simulink model "reguladores"  (R2019a)
settings: Solver=VariableStepAuto  StartTime=0.0  StopTime=10.0  RelTol=1e-3
undefined symbols (not defined in the file): Kregulador
settings Model: Creator=julia  LastModifiedBy=julia

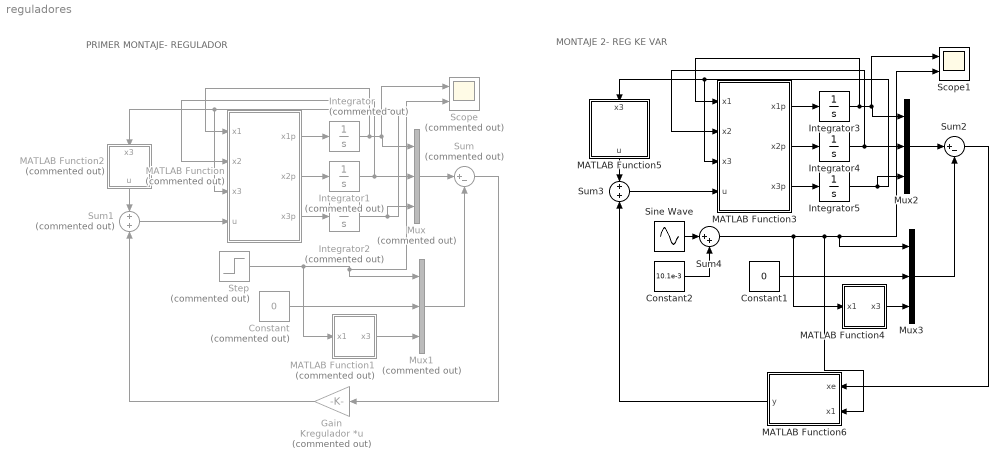
== system reguladores ==
  note: MONTAJE 2- REG KE VAR
  note: PRIMER MONTAJE- REGULADOR
  Constant : Constant  Commented=on  Value=0
  Constant1 : Constant  Value=0
  Constant2 : Constant  Value=10.1e-3
  Gain : Gain  Commented=on  Gain=Kregulador  Multiplication=Matrix(K*u)
  Integrator : Integrator  Commented=on  InitialCondition=5e-3
  Integrator1 : Integrator  Commented=on
  Integrator2 : Integrator  Commented=on
  Integrator3 : Integrator  InitialCondition=5e-3
  Integrator4 : Integrator
  Integrator5 : Integrator
  MATLAB Function : MATLAB Function  Commented=on  TreatAsAtomicUnit=on
  MATLAB Function1 : MATLAB Function  Commented=on  TreatAsAtomicUnit=on
  MATLAB Function2 : MATLAB Function  Commented=on  TreatAsAtomicUnit=on
  MATLAB Function3 : MATLAB Function  TreatAsAtomicUnit=on
  MATLAB Function4 : MATLAB Function  TreatAsAtomicUnit=on
  MATLAB Function5 : MATLAB Function  TreatAsAtomicUnit=on
  MATLAB Function6 : MATLAB Function  TreatAsAtomicUnit=on
  Mux : Mux  Commented=on  Inputs=3
  Mux1 : Mux  Commented=on  Inputs=3
  Mux2 : Mux  Inputs=3
  Mux3 : Mux  Inputs=3
  Scope : Scope  Commented=on  NumInputPorts=2
  Scope1 : Scope  NumInputPorts=2
  Sine Wave : Sin  Amplitude=10e-3  Frequency=2  Phase=3+pi/2  SampleTime=0
  Step : Step  Commented=on  Time=0  Before=5e-3  After=10e-3  SampleTime=0
  Sum : Sum  Commented=on  Inputs=|+-
  Sum1 : Sum  Commented=on  Inputs=+|+
  Sum2 : Sum  Inputs=|+-
  Sum3 : Sum  Inputs=+|+
  Sum4 : Sum  Inputs=|++
  wires:
  Sum2/1 -> MATLAB Function6/1(xe)
  Constant2/1 -> Sum4/2
  Sine Wave/1 -> Sum4/1
  MATLAB Function3/1(x1p) -> Integrator3/1
  MATLAB Function3/2(x2p) -> Integrator4/1
  MATLAB Function3/3(x3p) -> Integrator5/1
  Integrator3/1 -> MATLAB Function3/1(x1), Scope1/1, Mux2/1
  Integrator4/1 -> MATLAB Function3/2(x2), Mux2/2
  Integrator5/1 -> MATLAB Function5/1(x3), MATLAB Function3/3(x3), Mux2/3
  Mux2/1 -> Sum2/1
  Constant1/1 -> Mux3/2
  Sum4/1 -> MATLAB Function4/1(x1), Scope1/2, Mux3/1, MATLAB Function6/2(x1)
  MATLAB Function4/1(x3) -> Mux3/3
  Mux3/1 -> Sum2/2
  MATLAB Function6/1(y) -> Sum3/2
  Sum3/1 -> MATLAB Function3/4(u)
  MATLAB Function5/1(u) -> Sum3/1
  MATLAB Function2/1(u) -> Sum1/1
  Sum1/1 -> MATLAB Function/4(u)
  Gain/1 -> Sum1/2
  Sum/1 -> Gain/1
  Mux1/1 -> Sum/2
  MATLAB Function1/1(x3) -> Mux1/3
  Step/1 -> Mux1/1, Scope/2, MATLAB Function1/1(x1)
  Constant/1 -> Mux1/2
  Mux/1 -> Sum/1
  Integrator2/1 -> Mux/3, MATLAB Function/3(x3), MATLAB Function2/1(x3)
  Integrator1/1 -> Mux/2, MATLAB Function/2(x2)
  Integrator/1 -> Mux/1, Scope/1, MATLAB Function/1(x1)
  MATLAB Function/3(x3p) -> Integrator2/1
  MATLAB Function/2(x2p) -> Integrator1/1
  MATLAB Function/1(x1p) -> Integrator/1

== matlab function reguladores/MATLAB Function1 ==
  data: x1 input; x3 output
function x3  = fcn(x1)
c=1
m=0.1
L=0.01
r=1
g=9.81

x3=sqrt((m*g*x1)/c);

== matlab function reguladores/MATLAB Function ==
  data: x1 input; x1p output; x2 input; x3 input; x2p output; x3p output; u input
function [x1p,x2p,x3p] = fcn(x1,x2,x3,u)
c=0.1
m=0.01
L=100e-3
r=10
g=9.81

x1p=x2;
x2p=g-(c/m)*((x3^2)/x1);
x3p=-(r/L)*x3+(1/L)*u;

== matlab function reguladores/MATLAB Function2 ==
  data: x3 input; u output
function u  = fcn(x3)
c=1
m=0.1
L=0.01
r=1
g=9.81

u=r*x3;

== matlab function reguladores/MATLAB Function3 ==
  data: x1 input size=1; x1p output size=1; x2 input size=1; x3 input size=1; x2p output size=1; x3p output size=1; u input size=1
function [x1p,x2p,x3p] = planta(x1,x2,x3,u)
c=0.1
m=0.01
L=100e-3
r=10
g=9.81

x1p=x2;
x2p=g-(c/m)*((x3^2)/x1);
x3p=-(r/L)*x3+(1/L)*u;

== matlab function reguladores/MATLAB Function4 ==
  data: x1 input; x3 output
function x3  = fcn(x1)
c=1
m=0.1
L=0.01
r=1
g=9.81

x3=sqrt((m*g*x1)/c);

== matlab function reguladores/MATLAB Function5 ==
  data: x3 input size=1; u output size=1
function u  = u(x3)
c=1
m=0.1
L=0.01
r=1
g=9.81

u=r*x3;

== matlab function reguladores/MATLAB Function6 ==
  data: xe input size=3; x1 input size=1; y output size=1
function y = Kreg(xe,x1)

k1=-(3.638e-16*(7.1805e16*x1+7.5503e15))/(sqrt(0.981*x1));
k2=-(1.0204e-6*(3776000*x1+48069))/(sqrt(0.981*x1));
k3=-4.4;
K=[k1,k2,k3];

y = K*xe;
